simulink model "Voltage_and_Current_Measurement_STL__11032026"  (R2024b)
settings: Solver=VariableStepAuto  StartTime=0.0  StopTime=2.0  RelTol=1e-3  AbsTol=1e-3
libraries: spsRMSLib x4, spsPower3phInstantaneousLib x2, spsThreePhaseVIMeasurementLib x2, spsThreePhaseSeriesRLCLoadLib x1, spsThreePhaseSourceLib x1, spsThreePhaseSeriesRLCBranchLib x1, sps_lib x1
settings Model: Creator=cachu  LastModifiedBy=cachu
settings SolverCC: AutoScaleAbsTol=off  AlgebraicLoopSolver=TrustRegion  MaxZcPerStep=1
settings DebuggingCC: UnconnectedInputMsg=warning  UnconnectedOutputMsg=warning  UnconnectedLineMsg=warning  SymbolicDimsDataTypeCodeGenerationDiagnostic=none
settings ModelReferenceCC: EnableRefExpFcnMdlSchedulingChecks=on
settings SFSimCC: CustomCodeUndefinedFunction=UseInterfaceOnly
settings RTWCC: GPUComputeCapability=3.5  DLArmComputeVersion=19.05
settings SimscapeCC: SimscapeLogType=all  SimscapeLogSimulationStatistics=on  SimscapeLogDataHistory=10000

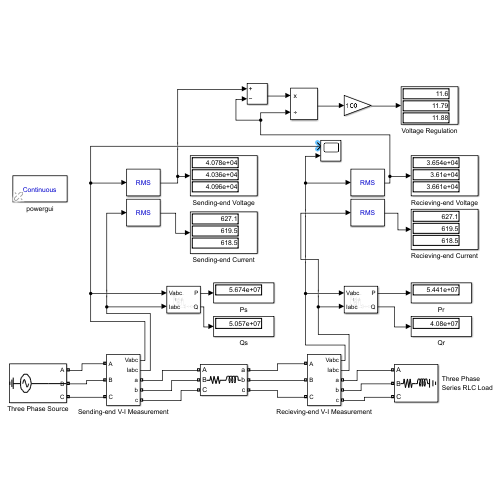
[thumbnail: Simulink's stored preview of the top-level diagram]
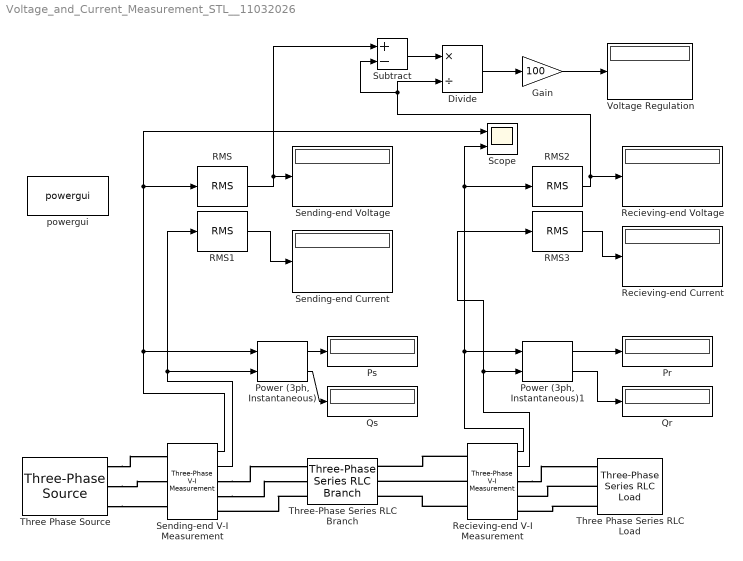
== system Voltage_and_Current_Measurement_STL__11032026 ==
  Divide : Product  Inputs=*/
  Gain : Gain  Gain=100
  "Power (3ph, Instantaneous)" : spsPower3phInstantaneousLib/Power (3ph, Instantaneous)
  "Power (3ph, Instantaneous)1" : spsPower3phInstantaneousLib/Power (3ph, Instantaneous)
  Pr : Display
  Ps : Display
  Qr : Display
  Qs : Display
  RMS{,1..3} (4 alike) : spsRMSLib/RMS  TrueRMS=on  Freq=60  RMSInit=120  Ts=0
  Recieving-end Current : Display
  Recieving-end V-I Measurement : spsThreePhaseVIMeasurementLib/Three-Phase V-I Measurement  VoltageMeasurement=phase-to-ground  SetLabelV=off  LabelV=Vabc  Vpu=off  VpuLL=off  CurrentMeasurement=yes  SetLabelI=off  LabelI=Iabc  Ipu=off  Pbase=100e6  Vbase=500e3  OutputType=Complex  PhasorSimulation=off  PSBequivalent=0
  Recieving-end Voltage : Display
  Scope : Scope  NumInputPorts=2
  Sending-end Current : Display
  Sending-end V-I Measurement : spsThreePhaseVIMeasurementLib/Three-Phase V-I Measurement  VoltageMeasurement=phase-to-ground  SetLabelV=off  LabelV=Vabc  Vpu=off  VpuLL=off  CurrentMeasurement=yes  SetLabelI=off  LabelI=Iabc  Ipu=off  Pbase=100e6  Vbase=500e3  OutputType=Complex  PhasorSimulation=off  PSBequivalent=0
  Sending-end Voltage : Display
  Subtract : Sum  Inputs=+-
  Three Phase Series RLC Load : spsThreePhaseSeriesRLCLoadLib/Three-Phase Series RLC Load  LConnTagsString=A|B|C  Configuration=Y (grounded)  NominalVoltage=64e3  Vabc=[1e3 1e3 1e3]  Vabcp=[1e3 1e3 1e3]  NominalFrequency=60  UnbalancedPower=off  ActivePower=56e6  InductivePower=42e6  CapacitivePower=0  Pabc=[10e3 9e3 11e3]  QLabc=[100 90 110]  QCabc=[100 90 110]  Pabcp=[10e3 9e3 11e3]  QLabcp=[100 90 110]  QCabcp=[100 90 110]  Measurements=None  LoadType=constant Z
  Three Phase Source : spsThreePhaseSourceLib/Three-Phase Source  InternalConnection=Yg  VoltagePhases=off  Voltage=70.5e3  PhaseAngle=0  Voltage_phases=[25e3 25e3 25e3]/sqrt(3)  PhaseAngles_phases=[0 -120 +120]  Frequency=60  NonIdealSource=off  SpecifyImpedance=on  Resistance=0.8929  Inductance=16.58e-3  ShortCircuitLevel=100e6  BaseVoltage=25e3  XRratio=7  BusType=swing  Pref=10e3  Qref=0  Prefabc=[10e3, 10e3, 10e3]  Qrefabc=[0, 0, 0]  Qmin=-inf  Qmax=inf
  Three-Phase Series RLC Branch : spsThreePhaseSeriesRLCBranchLib/Three-Phase Series RLC Branch  LConnTagsString=A|B|C  RConnTagsString=A|B|C  BranchType=RL  Resistance=2  Inductance=22.3e-3  Capacitance=1e-6  Measurements=None
  Voltage Regulation : Display
  powergui : sps_lib/powergui  Priority=1  SimulationMode=Continuous  SampleTime=50e-6  frequency=60  Iterations=50  frequencyindice=60  Pbase=100e6  ErrMax=1e-4  UnitsV=kV  UnitsW=MW  buscounter=0  FunctionMessages=off  echomessages=off  EnableUseOfTLC=off  CurrentSourceSwitches=off  DisableSnubberDevices=off  DisableRonSwitches=off  DisableVfSwitches=off  DisplayEquations=off  AutomaticDiscreteSolvers=off  SolverType=Tustin/Backward Euler (TBE)  Interpol=off  ExternalGateDelay=off  methode=off  Ts=100  x0status=blocks  SPID=on  SwTol=0  HookPort=off  NonlinearTolerance=1e-4  nMaxIteration=100  ContinueOnMaxIteration=off  RestoreLinks=warning  ResistiveCurrentMeasurement=off  Frange=[0:2:500]  Ylog=off  Xlog=on  ShowGrid=off  save=off  variable=ZData  structure=0  ZoomFFT=off  StartTime=0.0  cycles=1  DisplayStyle=1  fundamental=60  FreqAxis=off  MaxFrequency=1000  frequencyindicesteady=1  RmsSteady=1  display=off
  wires:
  Sending-end V-I Measurement/2 -> "Power (3ph, Instantaneous)"/2, RMS1/1
  Sending-end V-I Measurement/1 -> Scope/1, RMS/1, "Power (3ph, Instantaneous)"/1
  Recieving-end V-I Measurement/1 -> Scope/2, RMS2/1, "Power (3ph, Instantaneous)1"/1
  Recieving-end V-I Measurement/2 -> RMS3/1, "Power (3ph, Instantaneous)1"/2
  "Power (3ph, Instantaneous)"/1 -> Ps/1
  "Power (3ph, Instantaneous)"/2 -> Qs/1
  "Power (3ph, Instantaneous)1"/1 -> Pr/1
  "Power (3ph, Instantaneous)1"/2 -> Qr/1
  RMS/1 -> Subtract/1, Sending-end Voltage/1
  RMS1/1 -> Sending-end Current/1
  RMS3/1 -> Recieving-end Current/1
  RMS2/1 -> Divide/2, Subtract/2, Recieving-end Voltage/1
  Gain/1 -> Voltage Regulation/1
  Subtract/1 -> Divide/1
  Divide/1 -> Gain/1
  connections:
  Three Phase Source/RConn1 -- Sending-end V-I Measurement/LConn1
  Three Phase Source/RConn2 -- Sending-end V-I Measurement/LConn2
  Three Phase Source/RConn3 -- Sending-end V-I Measurement/LConn3
  Sending-end V-I Measurement/RConn1 -- Three-Phase Series RLC Branch/LConn1
  Sending-end V-I Measurement/RConn2 -- Three-Phase Series RLC Branch/LConn2
  Three-Phase Series RLC Branch/LConn3 -- Sending-end V-I Measurement/RConn3
  Recieving-end V-I Measurement/RConn1 -- Three Phase Series RLC Load/LConn1
  Recieving-end V-I Measurement/LConn1 -- Three-Phase Series RLC Branch/RConn1
  Recieving-end V-I Measurement/LConn2 -- Three-Phase Series RLC Branch/RConn2
  Recieving-end V-I Measurement/LConn3 -- Three-Phase Series RLC Branch/RConn3
  Three Phase Series RLC Load/LConn2 -- Recieving-end V-I Measurement/RConn2
  Three Phase Series RLC Load/LConn3 -- Recieving-end V-I Measurement/RConn3
